simulink model "Acceleration_Integrators"  (R2019b)
settings: Solver=VariableStepAuto  StartTime=0.0  StopTime=10.0  RelTol=1e-3
values from neighbouring files (symbols this model uses):
  A = [1 0; 1 0]    [test_kf_simple.m]
  B = [1; 0]    [test_kf_simple.m]
  C = [1 -1; 0 1]    [test_kf_simple.m]
undefined symbols (not defined in the file or in its folder): Add, Bdd, Cdd, Ddd
settings Model: Creator=thinhhoang  LastModifiedBy=thinhhoang

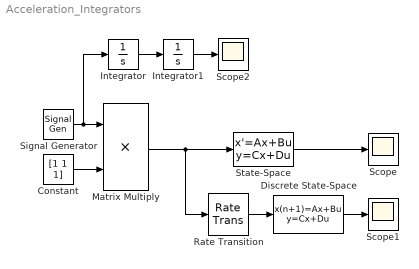
== system Acceleration_Integrators ==
  Constant : Constant  Value=[1 1 1]
  Discrete State-Space : DiscreteStateSpace  A=Add  B=Bdd  C=Cdd  D=Ddd  SampleTime=-1
  Integrator : Integrator
  Integrator1 : Integrator
  Matrix Multiply : Product
  Rate Transition : RateTransition  OutPortSampleTime=imuTs
  Scope : Scope
  Scope1 : Scope
  Scope2 : Scope
  Signal Generator : SignalGenerator  WaveForm=sawtooth  Units=rad/sec
  State-Space : StateSpace  A=A  B=B  C=C  D=zeros(3)  InitialCondition=0
  wires:
  State-Space/1 -> Scope/1
  Rate Transition/1 -> Discrete State-Space/1
  Discrete State-Space/1 -> Scope1/1
  Signal Generator/1 -> Integrator/1, Matrix Multiply/1
  Constant/1 -> Matrix Multiply/2
  Matrix Multiply/1 -> Rate Transition/1, State-Space/1
  Integrator/1 -> Integrator1/1
  Integrator1/1 -> Scope2/1
